simulink model "battery_fault_detection_model"  (R2024a)
settings: Solver=VariableStepAuto  StartTime=0.0  StopTime=3000  RelTol=1e-3
undefined symbols (not defined in the file or in its folder): a1, a1_1, a1_2, a1_3, a1_4, A2, a2, A2_2, A2_3, A2_4, A2_5, b1, b1_1, b1_2, b1_3, b1_4, B2, B2_2, B2_3, B2_4, B2_5, C1, C2m, C2m_2, C2m_3, C2m_4, C2m_5, Cbat, Cell, D2, D2_2, D2_3, D2_4, D2_5, dOCV, OCV, P0, Qb, R, R1, SoC0, SOC_bp, Ts
libraries: simulink x8, dspstat3 x1
settings Model: Creator=mukir  LastModifiedBy=mukir
settings DataIOCC: ReturnWorkspaceOutputs=off

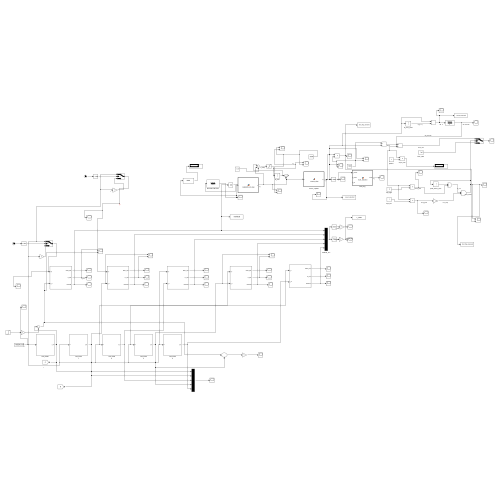
[thumbnail: Simulink's stored preview of the top-level diagram]
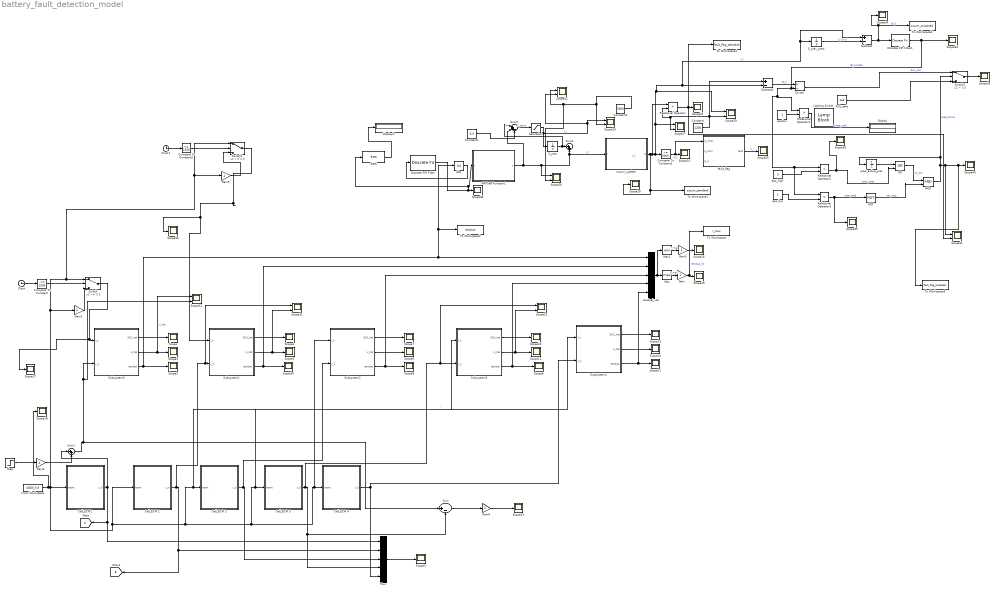
== system battery_fault_detection_model ==
  note: d_i
  note: d_i
  AND : Logic  IconShape=distinctive  AllPortsSameDT=off  OutDataTypeStr=boolean
  Abs : Abs  SaturateOnIntegerOverflow=off
  Cell_ECM 1 : Subsystem
  Cell_ECM 2 : Subsystem
  Cell_ECM 3 : Subsystem
  Cell_ECM 4 : Subsystem
  "Cell_ECM1 " : Subsystem
  Clock : Clock
  Clock1 : Clock
  Compare To Constant : simulink/Logic and Bit Operations/Compare To Constant  relop=<=  const=1500  OutDataTypeStr=boolean
  Compare To Constant1 : simulink/Logic and Bit Operations/Compare To Constant  relop=>=  const=3000  OutDataTypeStr=boolean
  Compare To Constant2 : simulink/Logic and Bit Operations/Compare To Constant  relop=<=  const=1500  OutDataTypeStr=boolean
  Constant : Constant  Value=1200
  Constant1 : Constant  Value=0.5
  Constant2 : Constant  Value=3000
  Discrete FIR Filter : DiscreteFir  Coefficients=(1/50)*ones(1,50)
  Discrete FIR Filter1 : DiscreteFir  Coefficients=ones(1,10)/10
  Display : Display
  Display2 : Display
  Divide : Product  Inputs=*/
  From Workspace : FromWorkspace  VariableName=UDDS_full  SampleTime=1
  Gain{,1..5} (6 alike) : Gain
  Goto : Goto  TagVisibility=global
  Lighting Switch : LampBlock  LabelPosition=Hide  Icon=LightingSwitch
  MATLAB Function1 : MATLAB Function  TreatAsAtomicUnit=on
  Max : MinMax  Function=max
  Max1 : MinMax
  Mux : Mux  Inputs=5
  NOT : Logic  Operator=NOT  IconShape=distinctive  AllPortsSameDT=off  OutDataTypeStr=boolean
  OR : Logic  Operator=OR  IconShape=distinctive  AllPortsSameDT=off  OutDataTypeStr=boolean
  RMS : dspstat3/RMS  run=off  directionMode=Each column  dimension=1  InputProcessing=Columns as channels (frame based)  reset_popup=None
  "RUL_safe " : Constant  Value=1e6
  Relational Operator : RelationalOperator  Operator=>  OutDataTypeStr=boolean  RndMeth=Simplest  InputSameDT=off
  Relational Operator1 : RelationalOperator  Operator=>  OutDataTypeStr=boolean  RndMeth=Simplest  InputSameDT=off
  Relational Operator2 : RelationalOperator  Operator=>  OutDataTypeStr=boolean  RndMeth=Simplest  InputSameDT=off
  Relational Operator3 : RelationalOperator  Operator=<  OutDataTypeStr=boolean  RndMeth=Simplest  InputSameDT=off
  "S_prev " : UnitDelay  SampleTime=-1  HasFrameUpgradeWarning=on
  S_prev_pred : UnitDelay  SampleTime=-1  HasFrameUpgradeWarning=on
  Saturation : Saturate  UpperLimit=inf  LowerLimit=0
  Scope{,1..11,13..18,20..21,23..25,28,30,33..40} (33 alike) : Scope
  Scope{12,19,22,26..27,29,31..32,41} (9 alike) : Scope  NumInputPorts=2
  Step : Step  Time=1500  After=0.02  SampleTime=0
  Subsystem1 : Subsystem
  Subsystem2 : Subsystem
  Subsystem3 : Subsystem
  Subsystem4 : Subsystem
  Subsystem5 : Subsystem
  Subtract : Sum  Inputs=+-
  Subtract1 : Sum  Inputs=+-
  Sum : Sum  Inputs=|+-
  Sum1 : Sum  Inputs=|++
  Sum2 : Sum  Inputs=|++
  Sum5 : Sum  Inputs=|++-
  Switch : Switch  Threshold=0.5  SaturateOnIntegerOverflow=off  InputSameDT=off
  Switch1 : Switch  Threshold=0.5  SaturateOnIntegerOverflow=off  InputSameDT=off
  Switch2 : Switch  Criteria=u2 > Threshold  Threshold=0.5  SaturateOnIntegerOverflow=off  InputSameDT=off
  To Workspace : ToWorkspace  VariableName=r_max  SaveFormat=Timeseries  SampleTime=-1
  To Workspace1 : ToWorkspace  VariableName=cusum_standard  SampleTime=-1
  To Workspace2 : ToWorkspace  VariableName=residual  SampleTime=-1
  To Workspace3 : ToWorkspace  VariableName=cusum_proposed  SaveFormat=Timeseries  SampleTime=-1
  To Workspace4 : ToWorkspace  VariableName=fault_flag_standard  SampleTime=-1
  To Workspace5 : ToWorkspace  VariableName=fault_flag_proposed  SampleTime=-1
  "cusum_update " : MATLAB Function  TreatAsAtomicUnit=on
  eps_high : Constant  Value=3
  eps_low : Constant
  "epsilon " : Constant
  fault_flag : MATLAB Function  TreatAsAtomicUnit=on
  "pred_active_prev " : UnitDelay  SampleTime=-1  HasFrameUpgradeWarning=on
  "residual_vec " : Mux  Inputs=5
  tag scope: B=global
  wires:
  Gain2/1 -> Sum1/2
  Step/1 -> Gain2/1
  Subsystem5/1(SOC_hat) -> Scope/1
  Subsystem5/3(residual) -> To Workspace2/1, Abs/1, "residual_vec "/1, Scope2/1
  Cell_ECM 1/1(y_k) -> Scope31/1, Subsystem1/2(y_k), [B], Mux/2
  Cell_ECM 2/1(y_k) -> Subsystem2/2(y_k), Mux/3
  Cell_ECM 4/1(y_k) -> Subsystem4/2(y_k), Mux/5
  Mux/1 -> Scope3/1
  Subsystem1/2(U_hat) -> Scope31/2, Scope5/1
  Subsystem1/1(SOC_hat) -> Scope4/1
  Subsystem2/3(residual) -> "residual_vec "/3, Scope8/1
  Subsystem2/1(SOC_hat) -> Scope7/1
  Subsystem3/3(residual) -> Scope6/1, "residual_vec "/4
  Subsystem3/1(SOC_hat) -> Scope10/1
  Subsystem4/3(residual) -> Scope21/1, "residual_vec "/5
  Subsystem4/2(U_hat) -> Scope14/1
  Subsystem4/1(SOC_hat) -> Scope13/1
  "residual_vec "/1 -> Max1/1, Max/1
  Max/1 -> Gain/1  "r_max"
  Clock/1 -> Compare To Constant/1
  Gain1/1 -> Switch/3
  Compare To Constant/1 -> Switch/2
  Max1/1 -> Gain3/1  "r_max"
  Gain3/1 -> Scope16/1
  Switch/1 -> Scope17/1, Subsystem5/1(I_k)
  Gain/1 -> Scope15/1, To Workspace/1  "residual_hp"
  Subsystem5/2(U_hat) -> Scope22/1, Scope1/1  "U_hat"
  Sum1/1 -> Scope22/2, Subsystem5/2(y_k), Sum/1
  Sum/1 -> Gain4/1
  Gain4/1 -> Scope23/1
  RMS/1 -> Display2/1
  Abs/1 -> Discrete FIR Filter/1
  Constant1/1 -> Sum5/3
  fault_flag/1(fault) -> Scope25/1  "s_i"
  Constant2/1 -> Scope19/2, Scope26/2, Scope32/1
  Sum5/1 -> Saturation/1  "S_temp"
  Compare To Constant1/1 -> fault_flag/1(d_umax), Scope24/1
  Constant/1 -> Subtract1/1, Scope29/2, Scope27/2, Relational Operator/2
  Discrete FIR Filter/1 -> RMS/1, MATLAB Function1/1(r), Scope36/1
  "S_prev "/1 -> Sum5/1, Sum2/1
  Saturation/1 -> Scope19/1, Scope32/2, "S_prev "/1  "s_i"
  Relational Operator/1 -> To Workspace4/1, Scope41/2, Scope37/1
  MATLAB Function1/1(s) -> Sum5/2, Scope26/1, "cusum_update "/1(r), Sum2/2  "s_i"
  "cusum_update "/1(S) -> To Workspace1/1, Scope28/1, Relational Operator/1, Subtract/1, S_prev_pred/1, Subtract1/2, Scope29/1, Scope27/1, Compare To Constant1/1  "s_i"
  "Cell_ECM1 "/1(y_k) -> Goto/1, Mux/1, Sum1/1
  Subsystem2/2(U_hat) -> Scope9/1
  Subsystem3/2(U_hat) -> Scope12/2, Scope11/1
  Cell_ECM 3/1(y_k) -> Scope12/1, Subsystem3/2(y_k), Sum/2, Mux/4
  Gain5/1 -> Switch1/3
  From Workspace/1 -> Scope18/1, Cell_ECM 1/1(Inport), Subsystem2/1(I_k), Cell_ECM 2/1(Inport), Subsystem3/1(I_k), Cell_ECM 3/1(Inport), Subsystem4/1(I_k), Cell_ECM 4/1(Inport), "Cell_ECM1 "/1(Inport), Switch1/1, Gain5/1, Switch/1, Gain1/1  "I"
  Compare To Constant2/1 -> Switch1/2
  Switch1/1 -> Subsystem1/1(I_k), Scope30/1
  Clock1/1 -> Compare To Constant2/1
  Subsystem1/3(residual) -> Scope20/1, "residual_vec "/2
  S_prev_pred/1 -> Subtract/2  "S_(k−1)"
  Subtract/1 -> Discrete FIR Filter1/1, To Workspace3/1, Scope34/1  "dS_k"
  Discrete FIR Filter1/1 -> Relational Operator3/1, Relational Operator2/1, Relational Operator1/1, Divide/2, Scope33/1  "dS_smooth"
  Subtract1/1 -> Divide/1  "dS_k"
  "epsilon "/1 -> Relational Operator1/2
  Relational Operator1/1 -> Display/1  "slope_valid"
  Divide/1 -> Switch2/1  "RUL_raw"
  "RUL_safe "/1 -> Switch2/3
  Switch2/1 -> Scope35/1
  eps_high/1 -> Relational Operator2/2
  Relational Operator2/1 -> Scope38/1, OR/2  "start_pred"
  eps_low/1 -> Relational Operator3/2
  Relational Operator3/1 -> Scope39/1, NOT/1  "stop_pred"
  "pred_active_prev "/1 -> OR/1
  OR/1 -> AND/1  "or_out"
  NOT/1 -> AND/2  "not_stop"
  AND/1 -> To Workspace5/1, Scope40/1, Scope41/1, Switch2/2, "pred_active_prev "/1  "pred_active"

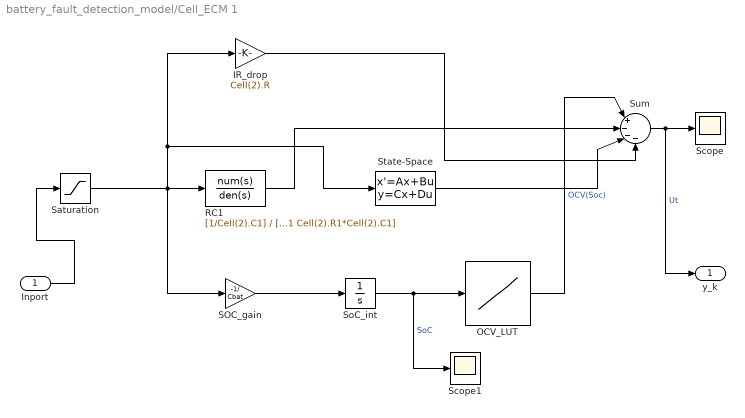
== system battery_fault_detection_model/Cell_ECM 1 ==
  Inport : Inport
  IR_drop : Gain  Gain=Cell(2).R
  OCV_LUT : Lookup_n-D  NumberOfTableDimensions=1  BreakpointsForDimension1=SOC_bp  Table=OCV  InternalRulePriority=Speed  RndMeth=Simplest
  RC1 : TransferFcn  Numerator=[1/Cell(2).C1]  Denominator=[1 Cell(2).R1*Cell(2).C1]
  SOC_gain : Gain  Gain=-1/ Cbat
  Saturation : Saturate  UpperLimit=12  LowerLimit=-6
  Scope : Scope
  Scope1 : Scope
  SoC_int : Integrator  InitialCondition=SoC0
  State-Space : StateSpace  A=A2_2  B=B2_2  C=C2m_2  D=D2_2  InitialCondition=0
  Sum : Sum  Inputs=|+---
  y_k : Outport
  wires:
  IR_drop/1 -> Sum/4
  RC1/1 -> Sum/2
  Saturation/1 -> SOC_gain/1, State-Space/1, IR_drop/1, RC1/1
  SOC_gain/1 -> SoC_int/1
  OCV_LUT/1 -> Sum/1  "OCV(Soc)"
  SoC_int/1 -> Scope1/1, OCV_LUT/1  "SoC"
  Sum/1 -> y_k/1, Scope/1  "Ut"
  State-Space/1 -> Sum/3
  Inport/1 -> Saturation/1

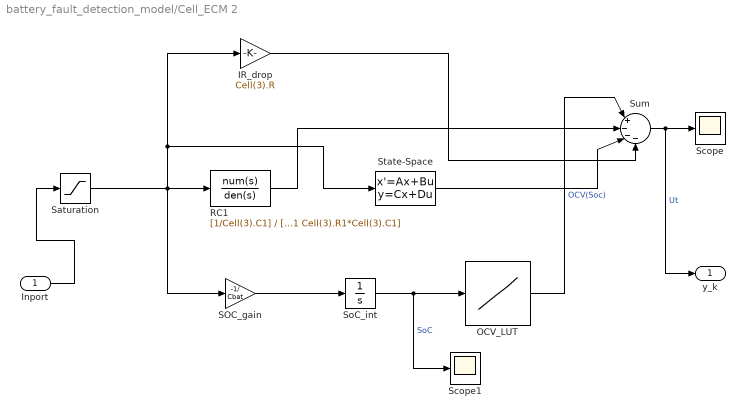
== system battery_fault_detection_model/Cell_ECM 2 ==
  Inport : Inport
  IR_drop : Gain  Gain=Cell(3).R
  OCV_LUT : Lookup_n-D  NumberOfTableDimensions=1  BreakpointsForDimension1=SOC_bp  Table=OCV  InternalRulePriority=Speed  RndMeth=Simplest
  RC1 : TransferFcn  Numerator=[1/Cell(3).C1]  Denominator=[1 Cell(3).R1*Cell(3).C1]
  SOC_gain : Gain  Gain=-1/ Cbat
  Saturation : Saturate  UpperLimit=12  LowerLimit=-6
  Scope : Scope
  Scope1 : Scope
  SoC_int : Integrator  InitialCondition=SoC0
  State-Space : StateSpace  A=A2_3  B=B2_3  C=C2m_3  D=D2_3  InitialCondition=0
  Sum : Sum  Inputs=|+---
  y_k : Outport
  wires:
  IR_drop/1 -> Sum/4
  RC1/1 -> Sum/2
  Saturation/1 -> SOC_gain/1, State-Space/1, IR_drop/1, RC1/1
  SOC_gain/1 -> SoC_int/1
  OCV_LUT/1 -> Sum/1  "OCV(Soc)"
  SoC_int/1 -> Scope1/1, OCV_LUT/1  "SoC"
  Sum/1 -> y_k/1, Scope/1  "Ut"
  State-Space/1 -> Sum/3
  Inport/1 -> Saturation/1

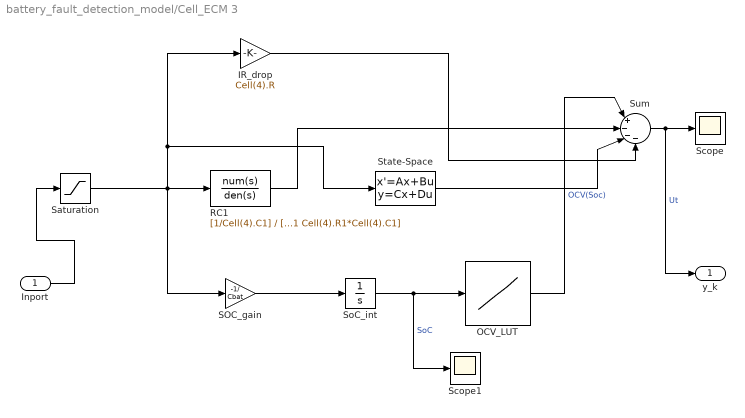
== system battery_fault_detection_model/Cell_ECM 3 ==
  Inport : Inport
  IR_drop : Gain  Gain=Cell(4).R
  OCV_LUT : Lookup_n-D  NumberOfTableDimensions=1  BreakpointsForDimension1=SOC_bp  Table=OCV  InternalRulePriority=Speed  RndMeth=Simplest
  RC1 : TransferFcn  Numerator=[1/Cell(4).C1]  Denominator=[1 Cell(4).R1*Cell(4).C1]
  SOC_gain : Gain  Gain=-1/ Cbat
  Saturation : Saturate  UpperLimit=12  LowerLimit=-6
  Scope : Scope
  Scope1 : Scope
  SoC_int : Integrator  InitialCondition=SoC0
  State-Space : StateSpace  A=A2_4  B=B2_4  C=C2m_4  D=D2_4  InitialCondition=0
  Sum : Sum  Inputs=|+---
  y_k : Outport
  wires:
  IR_drop/1 -> Sum/4
  RC1/1 -> Sum/2
  Saturation/1 -> SOC_gain/1, State-Space/1, IR_drop/1, RC1/1
  SOC_gain/1 -> SoC_int/1
  OCV_LUT/1 -> Sum/1  "OCV(Soc)"
  SoC_int/1 -> Scope1/1, OCV_LUT/1  "SoC"
  Sum/1 -> y_k/1, Scope/1  "Ut"
  State-Space/1 -> Sum/3
  Inport/1 -> Saturation/1

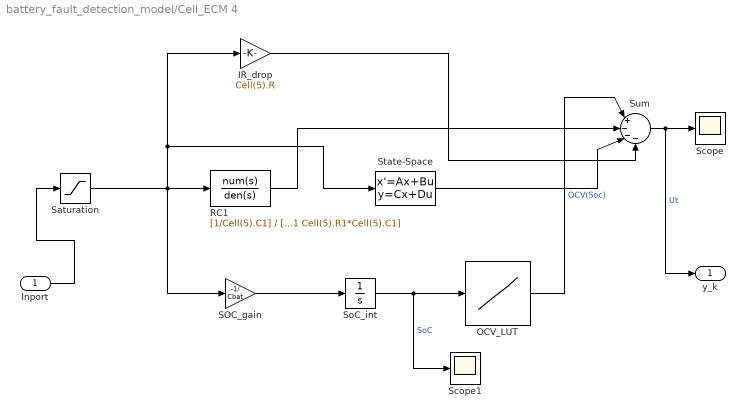
== system battery_fault_detection_model/Cell_ECM 4 ==
  Inport : Inport
  IR_drop : Gain  Gain=Cell(5).R
  OCV_LUT : Lookup_n-D  NumberOfTableDimensions=1  BreakpointsForDimension1=SOC_bp  Table=OCV  InternalRulePriority=Speed  RndMeth=Simplest
  RC1 : TransferFcn  Numerator=[1/Cell(5).C1]  Denominator=[1 Cell(5).R1*Cell(5).C1]
  SOC_gain : Gain  Gain=-1/ Cbat
  Saturation : Saturate  UpperLimit=12  LowerLimit=-6
  Scope : Scope
  Scope1 : Scope
  SoC_int : Integrator  InitialCondition=SoC0
  State-Space : StateSpace  A=A2_5  B=B2_5  C=C2m_5  D=D2_5  InitialCondition=0
  Sum : Sum  Inputs=|+---
  y_k : Outport
  wires:
  IR_drop/1 -> Sum/4
  RC1/1 -> Sum/2
  Saturation/1 -> SOC_gain/1, State-Space/1, IR_drop/1, RC1/1
  SOC_gain/1 -> SoC_int/1
  OCV_LUT/1 -> Sum/1  "OCV(Soc)"
  SoC_int/1 -> Scope1/1, OCV_LUT/1  "SoC"
  Sum/1 -> y_k/1, Scope/1  "Ut"
  State-Space/1 -> Sum/3
  Inport/1 -> Saturation/1

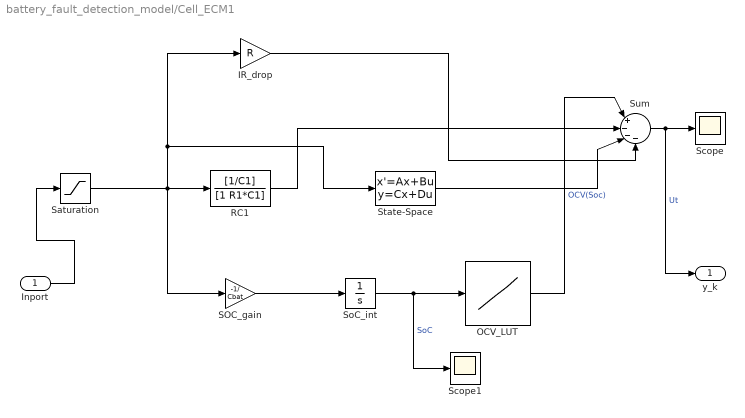
== system battery_fault_detection_model/Cell_ECM1  ==
  Inport : Inport
  IR_drop : Gain  Gain=R
  OCV_LUT : Lookup_n-D  NumberOfTableDimensions=1  BreakpointsForDimension1=SOC_bp  Table=OCV  InternalRulePriority=Speed  RndMeth=Simplest
  RC1 : TransferFcn  Numerator=[1/C1]  Denominator=[1 R1*C1]
  SOC_gain : Gain  Gain=-1/ Cbat
  Saturation : Saturate  UpperLimit=12  LowerLimit=-6
  Scope : Scope
  Scope1 : Scope
  SoC_int : Integrator  InitialCondition=SoC0
  State-Space : StateSpace  A=A2  B=B2  C=C2m  D=D2  InitialCondition=0
  Sum : Sum  Inputs=|+---
  y_k : Outport
  wires:
  IR_drop/1 -> Sum/4
  RC1/1 -> Sum/2
  Saturation/1 -> SOC_gain/1, State-Space/1, IR_drop/1, RC1/1
  SOC_gain/1 -> SoC_int/1
  OCV_LUT/1 -> Sum/1  "OCV(Soc)"
  SoC_int/1 -> Scope1/1, OCV_LUT/1  "SoC"
  Sum/1 -> y_k/1, Scope/1  "Ut"
  State-Space/1 -> Sum/3
  Inport/1 -> Saturation/1

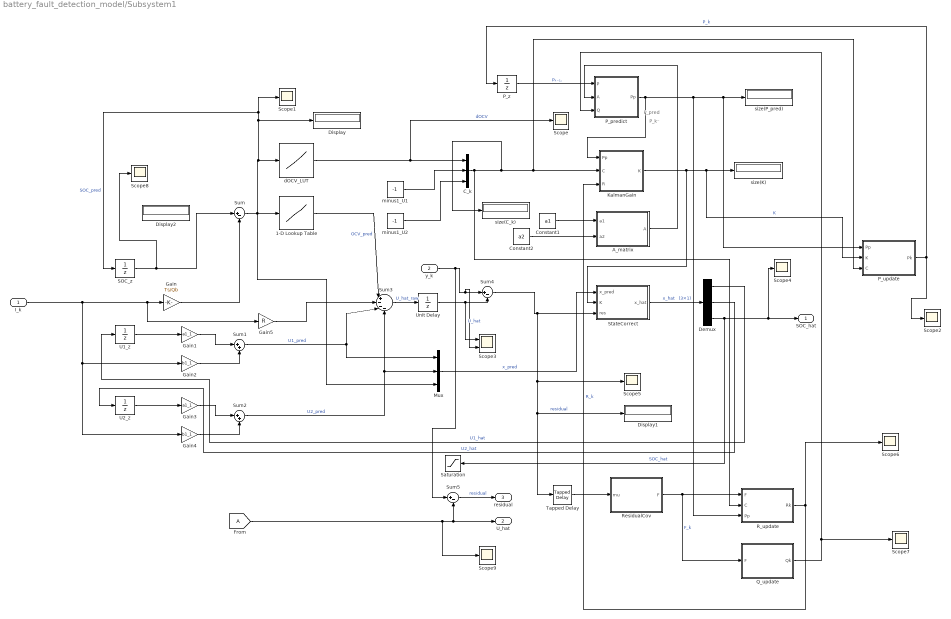
== system battery_fault_detection_model/Subsystem1 ==
  note: P_pred
  note: P_k⁻
  I_k : Inport
  y_k : Inport  Port=2
  1-D Lookup Table : Lookup_n-D  NumberOfTableDimensions=1  BreakpointsForDimension1=SOC_bp  Table=OCV  InternalRulePriority=Speed  RndMeth=Simplest
  A_matrix : MATLAB Function  TreatAsAtomicUnit=on
  "C_k " : Mux  Inputs=3
  Constant1 : Constant  Value=a1
  Constant2 : Constant  Value=a2
  Demux : Demux  Outputs=3
  Display : Display
  Display1 : Display
  Display2 : Display
  From : From  TagVisibility=global
  Gain : Gain  Gain=Ts/Qb
  Gain1 : Gain  Gain=a1_1
  Gain2 : Gain  Gain=b1_1
  Gain3 : Gain  Gain=a1_1
  Gain4 : Gain  Gain=b1_1
  Gain5 : Gain  Gain=R
  KalmanGain : MATLAB Function  TreatAsAtomicUnit=on
  Mux : Mux  Inputs=3
  P_predict : MATLAB Function  TreatAsAtomicUnit=on
  "P_update " : MATLAB Function  TreatAsAtomicUnit=on
  P_z : UnitDelay  InitialCondition=P0  SampleTime=-1  HasFrameUpgradeWarning=on
  Q_update : MATLAB Function  TreatAsAtomicUnit=on
  R_update : MATLAB Function  TreatAsAtomicUnit=on
  ResidualCov : MATLAB Function  TreatAsAtomicUnit=on
  SOC_z : UnitDelay  InitialCondition=0.6  SampleTime=-1  HasFrameUpgradeWarning=on
  Saturation : Saturate  UpperLimit=1  LowerLimit=0
  Scope{,1..2,4..9} (9 alike) : Scope
  Scope3 : Scope  NumInputPorts=2
  "StateCorrect " : MATLAB Function  TreatAsAtomicUnit=on
  Sum : Sum  Inputs=|+-
  Sum1 : Sum  Inputs=|++
  Sum2 : Sum  Inputs=|++
  Sum3 : Sum  Inputs=|+---
  Sum4 : Sum  Inputs=|+-
  Sum5 : Sum  Inputs=|+-
  Tapped Delay : simulink/Discrete/Tapped Delay  vinit=0.0  samptime=-1  NumDelays=20  DelayOrder=Newest  includeCurrent=on
  U1_z : UnitDelay  SampleTime=-1  HasFrameUpgradeWarning=on
  U2_z : UnitDelay  SampleTime=-1  HasFrameUpgradeWarning=on
  Unit Delay : UnitDelay  InitialCondition=3.33  SampleTime=-1  HasFrameUpgradeWarning=on
  "dOCV_LUT " : Lookup_n-D  NumberOfTableDimensions=1  BreakpointsForDimension1=SOC_bp  Table=dOCV  InternalRulePriority=Speed  RndMeth=Simplest
  minus1_U1 : Constant  Value=-1
  minus1_U2 : Constant  Value=-1
  size(C_k) : Display
  size(K) : Display
  size(P_pred) : Display
  SOC_hat : Outport
  U_hat : Outport  Port=2
  residual : Outport  Port=3
  wires:
  Gain/1 -> Sum/2
  Sum/1 -> Mux/3, Display/1, SOC_z/1, Scope1/1, "dOCV_LUT "/1, 1-D Lookup Table/1  "SOC_pred"
  U1_z/1 -> Gain1/1
  Gain1/1 -> Sum1/1
  Gain2/1 -> Sum1/2
  Sum1/1 -> Sum3/3, Mux/1  "U1_pred"
  Sum2/1 -> Mux/2, Sum3/4  "U2_pred"
  Gain4/1 -> Sum2/2
  U2_z/1 -> Gain3/1
  Gain3/1 -> Sum2/1
  1-D Lookup Table/1 -> Sum3/1  "OCV_pred"
  Gain5/1 -> Sum3/2
  Sum3/1 -> Unit Delay/1  "U_hat_raw"
  Unit Delay/1 -> Scope3/1, Sum4/2  "U_hat"
  y_k/1 -> Sum5/1, Scope3/2, Sum4/1
  Sum4/1 -> Scope5/1, Display1/1, Tapped Delay/1, "StateCorrect "/3(res)  "residual"
  "dOCV_LUT "/1 -> Scope/1, "C_k "/1  "dOCV"
  minus1_U1/1 -> "C_k "/2
  minus1_U2/1 -> "C_k "/3
  I_k/1 -> Gain4/1, Gain2/1, Gain5/1, Gain/1
  P_z/1 -> P_predict/1(P)  "Pₖ₋₁."
  P_predict/1(Pp) -> "P_update "/1(Pp), size(P_pred)/1, R_update/3(Pp), KalmanGain/1(Pp)
  "C_k "/1 -> size(C_k)/1, "P_update "/3(C), KalmanGain/2(C), R_update/2(C)
  Constant1/1 -> A_matrix/1(a1)
  Constant2/1 -> A_matrix/2(a2)
  A_matrix/1(A) -> P_predict/2(A)
  Q_update/1(Qk) -> Scope7/1, P_predict/3(Q)
  KalmanGain/1(K) -> "StateCorrect "/2(K), "P_update "/2(K), size(K)/1  "K"
  Mux/1 -> "StateCorrect "/1(x_pred)  "x_pred"
  "StateCorrect "/1(x_hat) -> Demux/1  "x_hat   (3×1)"
  Demux/1 -> U1_z/1  "U1_hat"
  Demux/2 -> U2_z/1  "U2_hat"
  Demux/3 -> Saturation/1, Scope4/1, SOC_hat/1  "SOC_hat"
  Tapped Delay/1 -> ResidualCov/1(mu)
  ResidualCov/1(F) -> Q_update/1(F), R_update/1(F)  "F_k"
  R_update/1(Rk) -> KalmanGain/3(R), Scope6/1  "R_k"
  "P_update "/1(Pk) -> Scope2/1, P_z/1  "P_k"
  SOC_z/1 -> Scope8/1, Sum/1
  From/1 -> Scope9/1, U_hat/1, Sum5/2
  Sum5/1 -> residual/1  "residual"

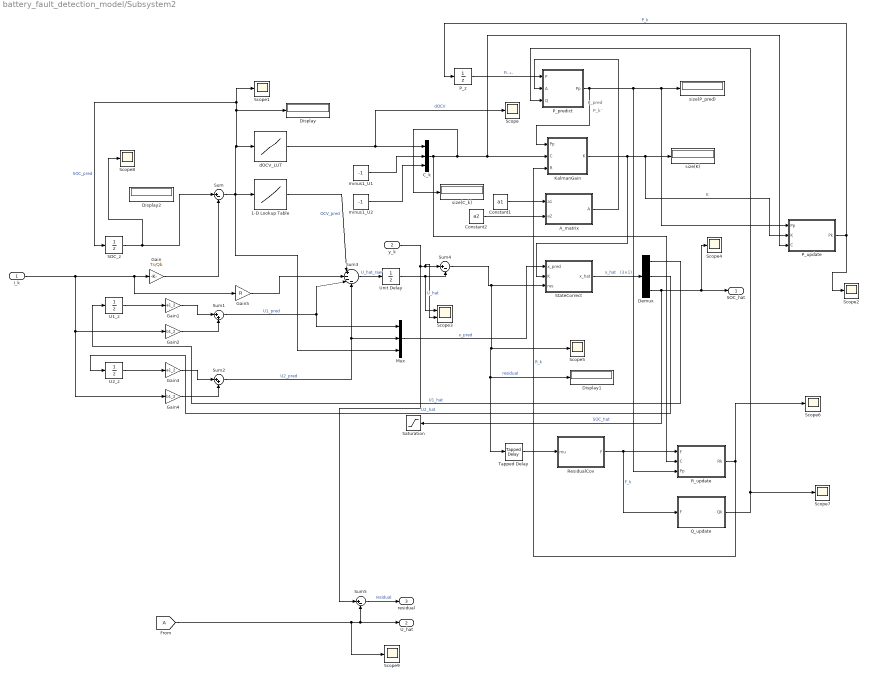
== system battery_fault_detection_model/Subsystem2 ==
  note: P_pred
  note: P_k⁻
  I_k : Inport
  y_k : Inport  Port=2
  1-D Lookup Table : Lookup_n-D  NumberOfTableDimensions=1  BreakpointsForDimension1=SOC_bp  Table=OCV  InternalRulePriority=Speed  RndMeth=Simplest
  A_matrix : MATLAB Function  TreatAsAtomicUnit=on
  "C_k " : Mux  Inputs=3
  Constant1 : Constant  Value=a1
  Constant2 : Constant  Value=a2
  Demux : Demux  Outputs=3
  Display : Display
  Display1 : Display
  Display2 : Display
  From : From  TagVisibility=global
  Gain : Gain  Gain=Ts/Qb
  Gain1 : Gain  Gain=a1_2
  Gain2 : Gain  Gain=b1_2
  Gain3 : Gain  Gain=a1_2
  Gain4 : Gain  Gain=b1_2
  Gain5 : Gain  Gain=R
  KalmanGain : MATLAB Function  TreatAsAtomicUnit=on
  Mux : Mux  Inputs=3
  P_predict : MATLAB Function  TreatAsAtomicUnit=on
  "P_update " : MATLAB Function  TreatAsAtomicUnit=on
  P_z : UnitDelay  InitialCondition=P0  SampleTime=-1  HasFrameUpgradeWarning=on
  Q_update : MATLAB Function  TreatAsAtomicUnit=on
  R_update : MATLAB Function  TreatAsAtomicUnit=on
  ResidualCov : MATLAB Function  TreatAsAtomicUnit=on
  SOC_z : UnitDelay  InitialCondition=0.6  SampleTime=-1  HasFrameUpgradeWarning=on
  Saturation : Saturate  UpperLimit=1  LowerLimit=0
  Scope{,1..2,4..9} (9 alike) : Scope
  Scope3 : Scope  NumInputPorts=2
  "StateCorrect " : MATLAB Function  TreatAsAtomicUnit=on
  Sum : Sum  Inputs=|+-
  Sum1 : Sum  Inputs=|++
  Sum2 : Sum  Inputs=|++
  Sum3 : Sum  Inputs=|+---
  Sum4 : Sum  Inputs=|+-
  Sum5 : Sum  Inputs=|+-
  Tapped Delay : simulink/Discrete/Tapped Delay  vinit=0.0  samptime=-1  NumDelays=20  DelayOrder=Newest  includeCurrent=on
  U1_z : UnitDelay  SampleTime=-1  HasFrameUpgradeWarning=on
  U2_z : UnitDelay  SampleTime=-1  HasFrameUpgradeWarning=on
  Unit Delay : UnitDelay  InitialCondition=3.33  SampleTime=-1  HasFrameUpgradeWarning=on
  "dOCV_LUT " : Lookup_n-D  NumberOfTableDimensions=1  BreakpointsForDimension1=SOC_bp  Table=dOCV  InternalRulePriority=Speed  RndMeth=Simplest
  minus1_U1 : Constant  Value=-1
  minus1_U2 : Constant  Value=-1
  size(C_k) : Display
  size(K) : Display
  size(P_pred) : Display
  SOC_hat : Outport
  U_hat : Outport  Port=2
  residual : Outport  Port=3
  wires:
  Gain/1 -> Sum/2
  Sum/1 -> Mux/3, Display/1, SOC_z/1, Scope1/1, "dOCV_LUT "/1, 1-D Lookup Table/1  "SOC_pred"
  U1_z/1 -> Gain1/1
  Gain1/1 -> Sum1/1
  Gain2/1 -> Sum1/2
  Sum1/1 -> Sum3/3, Mux/1  "U1_pred"
  Sum2/1 -> Mux/2, Sum3/4  "U2_pred"
  Gain4/1 -> Sum2/2
  U2_z/1 -> Gain3/1
  Gain3/1 -> Sum2/1
  1-D Lookup Table/1 -> Sum3/1  "OCV_pred"
  Gain5/1 -> Sum3/2
  Sum3/1 -> Unit Delay/1  "U_hat_raw"
  Unit Delay/1 -> Scope3/1, Sum4/2  "U_hat"
  Sum4/1 -> Scope5/1, Display1/1, Tapped Delay/1, "StateCorrect "/3(res)  "residual"
  "dOCV_LUT "/1 -> Scope/1, "C_k "/1  "dOCV"
  minus1_U1/1 -> "C_k "/2
  minus1_U2/1 -> "C_k "/3
  I_k/1 -> Gain4/1, Gain2/1, Gain5/1, Gain/1
  P_z/1 -> P_predict/1(P)  "Pₖ₋₁."
  P_predict/1(Pp) -> "P_update "/1(Pp), size(P_pred)/1, R_update/3(Pp), KalmanGain/1(Pp)
  "C_k "/1 -> size(C_k)/1, "P_update "/3(C), KalmanGain/2(C), R_update/2(C)
  Constant1/1 -> A_matrix/1(a1)
  Constant2/1 -> A_matrix/2(a2)
  A_matrix/1(A) -> P_predict/2(A)
  Q_update/1(Qk) -> Scope7/1, P_predict/3(Q)
  KalmanGain/1(K) -> "StateCorrect "/2(K), "P_update "/2(K), size(K)/1  "K"
  Mux/1 -> "StateCorrect "/1(x_pred)  "x_pred"
  "StateCorrect "/1(x_hat) -> Demux/1  "x_hat   (3×1)"
  Demux/1 -> U1_z/1  "U1_hat"
  Demux/2 -> U2_z/1  "U2_hat"
  Demux/3 -> Saturation/1, Scope4/1, SOC_hat/1  "SOC_hat"
  Tapped Delay/1 -> ResidualCov/1(mu)
  ResidualCov/1(F) -> Q_update/1(F), R_update/1(F)  "F_k"
  R_update/1(Rk) -> KalmanGain/3(R), Scope6/1  "R_k"
  "P_update "/1(Pk) -> Scope2/1, P_z/1  "P_k"
  SOC_z/1 -> Scope8/1, Sum/1
  Sum5/1 -> residual/1  "residual"
  From/1 -> Scope9/1, U_hat/1, Sum5/2
  y_k/1 -> Sum5/1, Scope3/2, Sum4/1

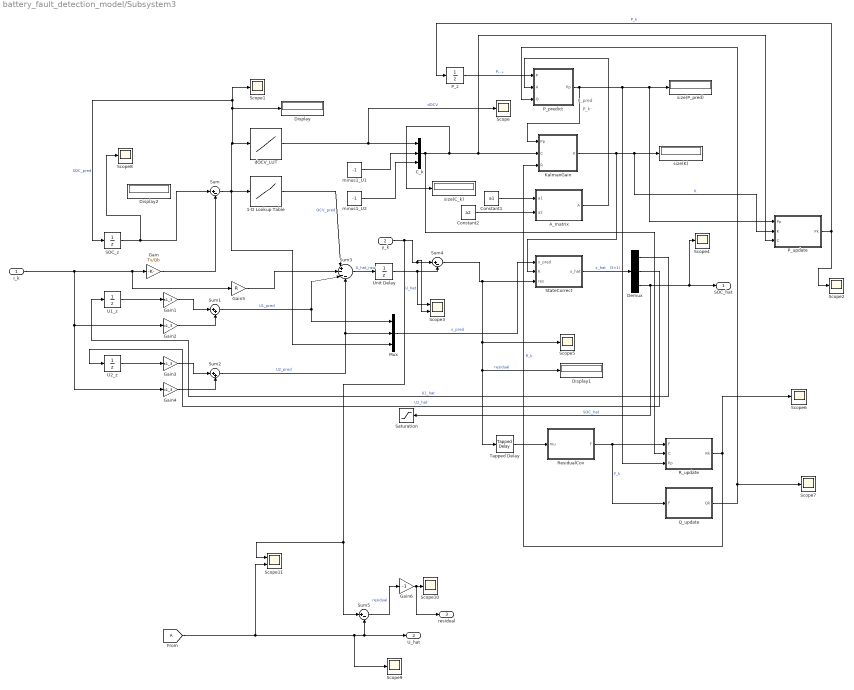
== system battery_fault_detection_model/Subsystem3 ==
  note: P_pred
  note: P_k⁻
  I_k : Inport
  y_k : Inport  Port=2
  1-D Lookup Table : Lookup_n-D  NumberOfTableDimensions=1  BreakpointsForDimension1=SOC_bp  Table=OCV  InternalRulePriority=Speed  RndMeth=Simplest
  A_matrix : MATLAB Function  TreatAsAtomicUnit=on
  "C_k " : Mux  Inputs=3
  Constant1 : Constant  Value=a1
  Constant2 : Constant  Value=a2
  Demux : Demux  Outputs=3
  Display : Display
  Display1 : Display
  Display2 : Display
  From : From  TagVisibility=global
  Gain : Gain  Gain=Ts/Qb
  Gain1 : Gain  Gain=a1_3
  Gain2 : Gain  Gain=b1_3
  Gain3 : Gain  Gain=a1_3
  Gain4 : Gain  Gain=b1_3
  Gain5 : Gain  Gain=R
  Gain6 : Gain  Gain=-1
  KalmanGain : MATLAB Function  TreatAsAtomicUnit=on
  Mux : Mux  Inputs=3
  P_predict : MATLAB Function  TreatAsAtomicUnit=on
  "P_update " : MATLAB Function  TreatAsAtomicUnit=on
  P_z : UnitDelay  InitialCondition=P0  SampleTime=-1  HasFrameUpgradeWarning=on
  Q_update : MATLAB Function  TreatAsAtomicUnit=on
  R_update : MATLAB Function  TreatAsAtomicUnit=on
  ResidualCov : MATLAB Function  TreatAsAtomicUnit=on
  SOC_z : UnitDelay  InitialCondition=0.6  SampleTime=-1  HasFrameUpgradeWarning=on
  Saturation : Saturate  UpperLimit=1  LowerLimit=0
  Scope{,1..2,4..10} (10 alike) : Scope
  Scope11 : Scope  NumInputPorts=2
  Scope3 : Scope  NumInputPorts=2
  "StateCorrect " : MATLAB Function  TreatAsAtomicUnit=on
  Sum : Sum  Inputs=|+-
  Sum1 : Sum  Inputs=|++
  Sum2 : Sum  Inputs=|++
  Sum3 : Sum  Inputs=|+---
  Sum4 : Sum  Inputs=|+-
  Sum5 : Sum  Inputs=|+-
  Tapped Delay : simulink/Discrete/Tapped Delay  vinit=0.0  samptime=-1  NumDelays=20  DelayOrder=Newest  includeCurrent=on
  U1_z : UnitDelay  SampleTime=-1  HasFrameUpgradeWarning=on
  U2_z : UnitDelay  SampleTime=-1  HasFrameUpgradeWarning=on
  Unit Delay : UnitDelay  InitialCondition=3.33  SampleTime=-1  HasFrameUpgradeWarning=on
  "dOCV_LUT " : Lookup_n-D  NumberOfTableDimensions=1  BreakpointsForDimension1=SOC_bp  Table=dOCV  InternalRulePriority=Speed  RndMeth=Simplest
  minus1_U1 : Constant  Value=-1
  minus1_U2 : Constant  Value=-1
  size(C_k) : Display
  size(K) : Display
  size(P_pred) : Display
  SOC_hat : Outport
  U_hat : Outport  Port=2
  residual : Outport  Port=3
  wires:
  Gain/1 -> Sum/2
  Sum/1 -> Mux/3, Display/1, SOC_z/1, Scope1/1, "dOCV_LUT "/1, 1-D Lookup Table/1  "SOC_pred"
  U1_z/1 -> Gain1/1
  Gain1/1 -> Sum1/1
  Gain2/1 -> Sum1/2
  Sum1/1 -> Sum3/3, Mux/1  "U1_pred"
  Sum2/1 -> Mux/2, Sum3/4  "U2_pred"
  Gain4/1 -> Sum2/2
  U2_z/1 -> Gain3/1
  Gain3/1 -> Sum2/1
  1-D Lookup Table/1 -> Sum3/1  "OCV_pred"
  Gain5/1 -> Sum3/2
  Sum3/1 -> Unit Delay/1  "U_hat_raw"
  Unit Delay/1 -> Scope3/1, Sum4/2  "U_hat"
  Sum4/1 -> Scope5/1, Display1/1, Tapped Delay/1, "StateCorrect "/3(res)  "residual"
  "dOCV_LUT "/1 -> Scope/1, "C_k "/1  "dOCV"
  minus1_U1/1 -> "C_k "/2
  minus1_U2/1 -> "C_k "/3
  I_k/1 -> Gain4/1, Gain2/1, Gain5/1, Gain/1
  P_z/1 -> P_predict/1(P)  "Pₖ₋₁."
  P_predict/1(Pp) -> "P_update "/1(Pp), size(P_pred)/1, R_update/3(Pp), KalmanGain/1(Pp)
  "C_k "/1 -> size(C_k)/1, "P_update "/3(C), KalmanGain/2(C), R_update/2(C)
  Constant1/1 -> A_matrix/1(a1)
  Constant2/1 -> A_matrix/2(a2)
  A_matrix/1(A) -> P_predict/2(A)
  Q_update/1(Qk) -> Scope7/1, P_predict/3(Q)
  KalmanGain/1(K) -> "StateCorrect "/2(K), "P_update "/2(K), size(K)/1  "K"
  Mux/1 -> "StateCorrect "/1(x_pred)  "x_pred"
  "StateCorrect "/1(x_hat) -> Demux/1  "x_hat   (3×1)"
  Demux/1 -> U1_z/1  "U1_hat"
  Demux/2 -> U2_z/1  "U2_hat"
  Demux/3 -> Saturation/1, Scope4/1, SOC_hat/1  "SOC_hat"
  Tapped Delay/1 -> ResidualCov/1(mu)
  ResidualCov/1(F) -> Q_update/1(F), R_update/1(F)  "F_k"
  R_update/1(Rk) -> KalmanGain/3(R), Scope6/1  "R_k"
  "P_update "/1(Pk) -> Scope2/1, P_z/1  "P_k"
  SOC_z/1 -> Scope8/1, Sum/1
  y_k/1 -> Scope11/1, Sum5/1, Scope3/2, Sum4/1
  Sum5/1 -> Gain6/1  "residual"
  From/1 -> Scope9/1, U_hat/1, Sum5/2, Scope11/2
  Gain6/1 -> residual/1, Scope10/1

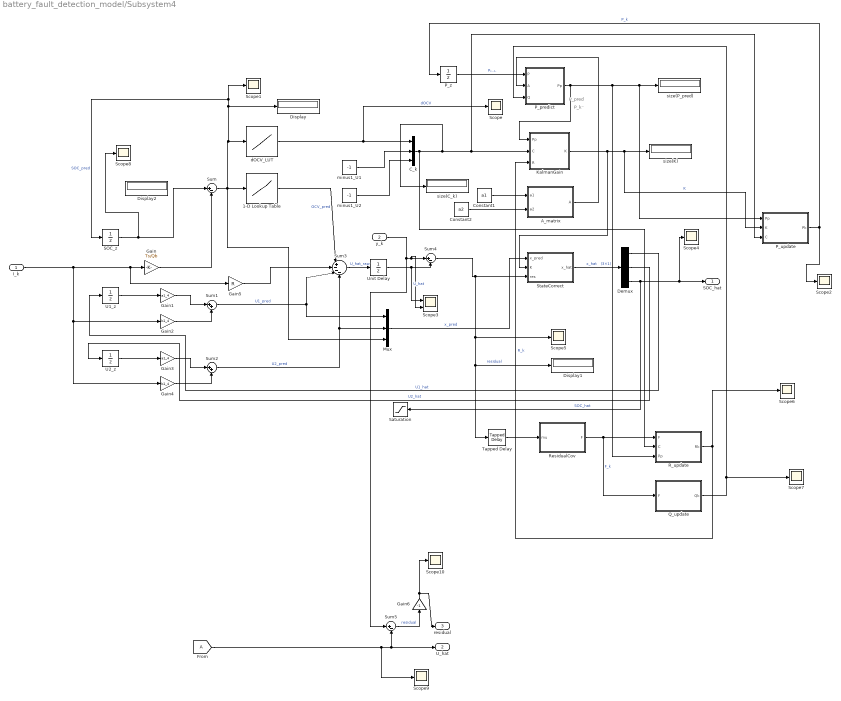
== system battery_fault_detection_model/Subsystem4 ==
  note: P_pred
  note: P_k⁻
  I_k : Inport
  y_k : Inport  Port=2
  1-D Lookup Table : Lookup_n-D  NumberOfTableDimensions=1  BreakpointsForDimension1=SOC_bp  Table=OCV  InternalRulePriority=Speed  RndMeth=Simplest
  A_matrix : MATLAB Function  TreatAsAtomicUnit=on
  "C_k " : Mux  Inputs=3
  Constant1 : Constant  Value=a1
  Constant2 : Constant  Value=a2
  Demux : Demux  Outputs=3
  Display : Display
  Display1 : Display
  Display2 : Display
  From : From  TagVisibility=global
  Gain : Gain  Gain=Ts/Qb
  Gain1 : Gain  Gain=a1_4
  Gain2 : Gain  Gain=b1_4
  Gain3 : Gain  Gain=a1_4
  Gain4 : Gain  Gain=b1_4
  Gain5 : Gain  Gain=R
  Gain6 : Gain  Gain=-1
  KalmanGain : MATLAB Function  TreatAsAtomicUnit=on
  Mux : Mux  Inputs=3
  P_predict : MATLAB Function  TreatAsAtomicUnit=on
  "P_update " : MATLAB Function  TreatAsAtomicUnit=on
  P_z : UnitDelay  InitialCondition=P0  SampleTime=-1  HasFrameUpgradeWarning=on
  Q_update : MATLAB Function  TreatAsAtomicUnit=on
  R_update : MATLAB Function  TreatAsAtomicUnit=on
  ResidualCov : MATLAB Function  TreatAsAtomicUnit=on
  SOC_z : UnitDelay  InitialCondition=0.6  SampleTime=-1  HasFrameUpgradeWarning=on
  Saturation : Saturate  UpperLimit=1  LowerLimit=0
  Scope{,1..2,4..10} (10 alike) : Scope
  Scope3 : Scope  NumInputPorts=2
  "StateCorrect " : MATLAB Function  TreatAsAtomicUnit=on
  Sum : Sum  Inputs=|+-
  Sum1 : Sum  Inputs=|++
  Sum2 : Sum  Inputs=|++
  Sum3 : Sum  Inputs=|+---
  Sum4 : Sum  Inputs=|+-
  Sum5 : Sum  Inputs=|+-
  Tapped Delay : simulink/Discrete/Tapped Delay  vinit=0.0  samptime=-1  NumDelays=20  DelayOrder=Newest  includeCurrent=on
  U1_z : UnitDelay  SampleTime=-1  HasFrameUpgradeWarning=on
  U2_z : UnitDelay  SampleTime=-1  HasFrameUpgradeWarning=on
  Unit Delay : UnitDelay  InitialCondition=3.33  SampleTime=-1  HasFrameUpgradeWarning=on
  "dOCV_LUT " : Lookup_n-D  NumberOfTableDimensions=1  BreakpointsForDimension1=SOC_bp  Table=dOCV  InternalRulePriority=Speed  RndMeth=Simplest
  minus1_U1 : Constant  Value=-1
  minus1_U2 : Constant  Value=-1
  size(C_k) : Display
  size(K) : Display
  size(P_pred) : Display
  SOC_hat : Outport
  U_hat : Outport  Port=2
  residual : Outport  Port=3
  wires:
  Gain/1 -> Sum/2
  Sum/1 -> Mux/3, Display/1, SOC_z/1, Scope1/1, "dOCV_LUT "/1, 1-D Lookup Table/1  "SOC_pred"
  U1_z/1 -> Gain1/1
  Gain1/1 -> Sum1/1
  Gain2/1 -> Sum1/2
  Sum1/1 -> Sum3/3, Mux/1  "U1_pred"
  Sum2/1 -> Mux/2, Sum3/4  "U2_pred"
  Gain4/1 -> Sum2/2
  U2_z/1 -> Gain3/1
  Gain3/1 -> Sum2/1
  1-D Lookup Table/1 -> Sum3/1  "OCV_pred"
  Gain5/1 -> Sum3/2
  Sum3/1 -> Unit Delay/1  "U_hat_raw"
  Unit Delay/1 -> Scope3/1, Sum4/2  "U_hat"
  Sum4/1 -> Scope5/1, Display1/1, Tapped Delay/1, "StateCorrect "/3(res)  "residual"
  "dOCV_LUT "/1 -> Scope/1, "C_k "/1  "dOCV"
  minus1_U1/1 -> "C_k "/2
  minus1_U2/1 -> "C_k "/3
  I_k/1 -> Gain4/1, Gain2/1, Gain5/1, Gain/1
  P_z/1 -> P_predict/1(P)  "Pₖ₋₁."
  P_predict/1(Pp) -> "P_update "/1(Pp), size(P_pred)/1, R_update/3(Pp), KalmanGain/1(Pp)
  "C_k "/1 -> size(C_k)/1, "P_update "/3(C), KalmanGain/2(C), R_update/2(C)
  Constant1/1 -> A_matrix/1(a1)
  Constant2/1 -> A_matrix/2(a2)
  A_matrix/1(A) -> P_predict/2(A)
  Q_update/1(Qk) -> Scope7/1, P_predict/3(Q)
  KalmanGain/1(K) -> "StateCorrect "/2(K), "P_update "/2(K), size(K)/1  "K"
  Mux/1 -> "StateCorrect "/1(x_pred)  "x_pred"
  "StateCorrect "/1(x_hat) -> Demux/1  "x_hat   (3×1)"
  Demux/1 -> U1_z/1  "U1_hat"
  Demux/2 -> U2_z/1  "U2_hat"
  Demux/3 -> Saturation/1, Scope4/1, SOC_hat/1  "SOC_hat"
  Tapped Delay/1 -> ResidualCov/1(mu)
  ResidualCov/1(F) -> Q_update/1(F), R_update/1(F)  "F_k"
  R_update/1(Rk) -> KalmanGain/3(R), Scope6/1  "R_k"
  "P_update "/1(Pk) -> Scope2/1, P_z/1  "P_k"
  SOC_z/1 -> Scope8/1, Sum/1
  y_k/1 -> Sum5/1, Scope3/2, Sum4/1
  Sum5/1 -> Gain6/1  "residual"
  From/1 -> Scope9/1, U_hat/1, Sum5/2
  Gain6/1 -> residual/1, Scope10/1

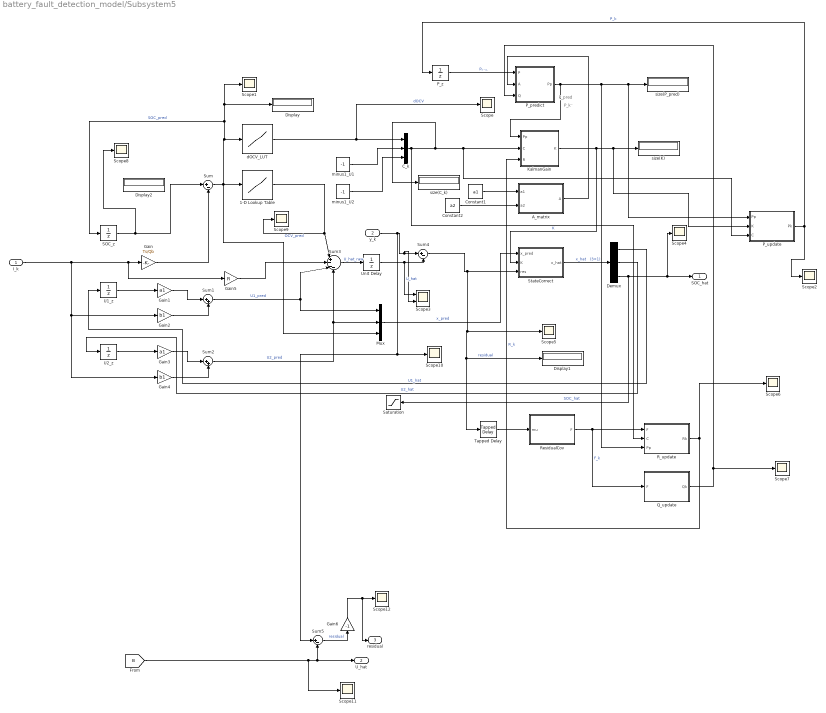
== system battery_fault_detection_model/Subsystem5 ==
  note: P_pred
  note: P_k⁻
  I_k : Inport
  y_k : Inport  Port=2
  1-D Lookup Table : Lookup_n-D  NumberOfTableDimensions=1  BreakpointsForDimension1=SOC_bp  Table=OCV  InternalRulePriority=Speed  RndMeth=Simplest
  A_matrix : MATLAB Function  TreatAsAtomicUnit=on
  "C_k " : Mux  Inputs=3
  Constant1 : Constant  Value=a1
  Constant2 : Constant  Value=a2
  Demux : Demux  Outputs=3
  Display : Display
  Display1 : Display
  Display2 : Display
  Gain : Gain  Gain=Ts/Qb
  Gain1 : Gain  Gain=a1
  Gain2 : Gain  Gain=b1
  Gain3 : Gain  Gain=a1
  Gain4 : Gain  Gain=b1
  Gain5 : Gain  Gain=R
  Gain6 : Gain  Gain=-1
  KalmanGain : MATLAB Function  TreatAsAtomicUnit=on
  Mux : Mux  Inputs=3
  P_predict : MATLAB Function  TreatAsAtomicUnit=on
  "P_update " : MATLAB Function  TreatAsAtomicUnit=on
  P_z : UnitDelay  InitialCondition=P0  SampleTime=-1  HasFrameUpgradeWarning=on
  Q_update : MATLAB Function  TreatAsAtomicUnit=on
  R_update : MATLAB Function  TreatAsAtomicUnit=on
  ResidualCov : MATLAB Function  TreatAsAtomicUnit=on
  SOC_z : UnitDelay  InitialCondition=0.6  SampleTime=-1  HasFrameUpgradeWarning=on
  Saturation : Saturate  UpperLimit=1  LowerLimit=0
  Scope{,1..2,4..12} (12 alike) : Scope
  Scope3 : Scope  NumInputPorts=2
  "StateCorrect " : MATLAB Function  TreatAsAtomicUnit=on
  Sum : Sum  Inputs=|+-
  Sum1 : Sum  Inputs=|++
  Sum2 : Sum  Inputs=|++
  Sum3 : Sum  Inputs=|+---
  Sum4 : Sum  Inputs=|+-
  Sum5 : Sum  Inputs=|+-
  Tapped Delay : simulink/Discrete/Tapped Delay  vinit=0.0  samptime=-1  NumDelays=20  DelayOrder=Newest  includeCurrent=on
  U1_z : UnitDelay  SampleTime=-1  HasFrameUpgradeWarning=on
  U2_z : UnitDelay  SampleTime=-1  HasFrameUpgradeWarning=on
  Unit Delay : UnitDelay  InitialCondition=3.32  SampleTime=-1  HasFrameUpgradeWarning=on
  "dOCV_LUT " : Lookup_n-D  NumberOfTableDimensions=1  BreakpointsForDimension1=SOC_bp  Table=dOCV  InternalRulePriority=Speed  RndMeth=Simplest
  minus1_U1 : Constant  Value=-1
  minus1_U2 : Constant  Value=-1
  size(C_k) : Display
  size(K) : Display
  size(P_pred) : Display
  SOC_hat : Outport
  U_hat : Outport  Port=2
  residual : Outport  Port=3
  wires:
  Gain/1 -> Sum/2
  Sum/1 -> Mux/3, SOC_z/1, Display/1, Scope1/1, "dOCV_LUT "/1, 1-D Lookup Table/1  "SOC_pred"
  U1_z/1 -> Gain1/1
  Gain1/1 -> Sum1/1
  Gain2/1 -> Sum1/2
  Sum1/1 -> Sum3/3, Mux/1  "U1_pred"
  Sum2/1 -> Mux/2, Sum3/4  "U2_pred"
  Gain4/1 -> Sum2/2
  U2_z/1 -> Gain3/1
  Gain3/1 -> Sum2/1
  1-D Lookup Table/1 -> Scope9/1, Sum3/1  "OCV_pred"
  Gain5/1 -> Sum3/2
  Sum3/1 -> Unit Delay/1  "U_hat_raw"
  Unit Delay/1 -> Scope3/1, Sum4/2  "U_hat"
  Sum4/1 -> Scope5/1, Display1/1, Tapped Delay/1, "StateCorrect "/3(res)  "residual"
  "dOCV_LUT "/1 -> Scope/1, "C_k "/1  "dOCV"
  minus1_U1/1 -> "C_k "/2
  minus1_U2/1 -> "C_k "/3
  I_k/1 -> Gain4/1, Gain2/1, Gain5/1, Gain/1
  P_z/1 -> P_predict/1(P)  "Pₖ₋₁."
  P_predict/1(Pp) -> "P_update "/1(Pp), size(P_pred)/1, R_update/3(Pp), KalmanGain/1(Pp)
  "C_k "/1 -> size(C_k)/1, "P_update "/3(C), KalmanGain/2(C), R_update/2(C)
  Constant1/1 -> A_matrix/1(a1)
  Constant2/1 -> A_matrix/2(a2)
  A_matrix/1(A) -> P_predict/2(A)
  Q_update/1(Qk) -> Scope7/1, P_predict/3(Q)
  KalmanGain/1(K) -> "StateCorrect "/2(K), "P_update "/2(K), size(K)/1  "K"
  Mux/1 -> "StateCorrect "/1(x_pred)  "x_pred"
  "StateCorrect "/1(x_hat) -> Demux/1  "x_hat   (3×1)"
  Demux/1 -> U1_z/1  "U1_hat"
  Demux/2 -> U2_z/1  "U2_hat"
  Demux/3 -> Saturation/1, Scope4/1, SOC_hat/1  "SOC_hat"
  Tapped Delay/1 -> ResidualCov/1(mu)
  ResidualCov/1(F) -> Q_update/1(F), R_update/1(F)  "F_k"
  R_update/1(Rk) -> KalmanGain/3(R), Scope6/1  "R_k"
  "P_update "/1(Pk) -> P_z/1, Scope2/1  "P_k"
  SOC_z/1 -> Scope8/1, Sum/1
  Sum5/1 -> Gain6/1  "residual"
  y_k/1 -> Scope10/1, Sum5/1, Scope3/2, Sum4/1
  [B] -> Scope11/1, U_hat/1, Sum5/2
  Gain6/1 -> residual/1, Scope12/1

== matlab function battery_fault_detection_model/Subsystem1/P_update  ==
  data: Pp input; Pk output; K input; C input
function Pk = P_update(Pp, K, C)
% Updated covariance: Pk = (I - K*C) * Pp
C = reshape(C,1,3);
I = eye(3);
Pk = (I - K*C) * Pp;
end

== matlab function battery_fault_detection_model/Subsystem1/Q_update ==
  data: F input; Qk output
function Qk = Q_update(F)
Qk = diag([0, 0, F]);   % 3×3 matrix
end

== matlab function battery_fault_detection_model/Subsystem5/P_predict ==
  data: P input; Pp output; A input; Q input
function Pp = P_predict(P, A, Q)
Pp = A*P*A' + Q;
end

== matlab function battery_fault_detection_model/Subsystem1/R_update ==
  data: F input; Rk output; C input; Pp input
function Rk = R_update(F, C, Pp)
C = reshape(C,1,3);
Rk = F + C*Pp*C';
end

== matlab function battery_fault_detection_model/Subsystem1/ResidualCov ==
  data: mu input; F output
function F = ResidualCov(mu)
mu = mu(:);              % force column vector
N  = length(mu);
F  = sum(mu.^2)/(N-1);   % scalar variance
end

== matlab function battery_fault_detection_model/Subsystem1/StateCorrect  ==
  data: x_pred input; x_hat output; K input; res input
function x_hat = StateCorrect(x_pred, K, res)
x_hat = x_pred + K * res;
end

== matlab function battery_fault_detection_model/Subsystem2/A_matrix ==
  data: a1 input; A output; a2 input
function A = A_matrix(a1, a2)
A = [a1 0  0;
     0  a2 0;
     0  0  1];
end

== matlab function battery_fault_detection_model/Subsystem2/KalmanGain ==
  data: Pp input; K output; C input; R input
function K = KalmanGain(Pp, C, R)
% Force dimensions explicitly
C = reshape(C, 1, 3);   % 1×3 row vector

S = C*Pp*C' + R;        % scalar
K = (Pp*C') / S;        % 3×1
end

== matlab function battery_fault_detection_model/Subsystem2/P_predict ==
  data: P input; Pp output; A input; Q input
function Pp = P_predict(P, A, Q)
Pp = A*P*A' + Q;
end

== matlab function battery_fault_detection_model/Subsystem2/P_update  ==
  data: Pp input; Pk output; K input; C input
function Pk = P_update(Pp, K, C)
% Updated covariance: Pk = (I - K*C) * Pp
C = reshape(C,1,3);
I = eye(3);
Pk = (I - K*C) * Pp;
end

== matlab function battery_fault_detection_model/Subsystem2/Q_update ==
  data: F input; Qk output
function Qk = Q_update(F)
Qk = diag([0, 0, F]);   % 3×3 matrix
end

== matlab function battery_fault_detection_model/Subsystem2/R_update ==
  data: F input; Rk output; C input; Pp input
function Rk = R_update(F, C, Pp)
C = reshape(C,1,3);
Rk = F + C*Pp*C';
end

== matlab function battery_fault_detection_model/Subsystem2/ResidualCov ==
  data: mu input; F output
function F = ResidualCov(mu)
mu = mu(:);              % force column vector
N  = length(mu);
F  = sum(mu.^2)/(N-1);   % scalar variance
end

== matlab function battery_fault_detection_model/Subsystem2/StateCorrect  ==
  data: x_pred input; x_hat output; K input; res input
function x_hat = StateCorrect(x_pred, K, res)
x_hat = x_pred + K * res;
end

== matlab function battery_fault_detection_model/Subsystem5/A_matrix ==
  data: a1 input; A output; a2 input
function A = A_matrix(a1, a2)
A = [a1 0  0;
     0  a2 0;
     0  0  1];
end

== matlab function battery_fault_detection_model/Subsystem3/A_matrix ==
  data: a1 input; A output; a2 input
function A = A_matrix(a1, a2)
A = [a1 0  0;
     0  a2 0;
     0  0  1];
end

== matlab function battery_fault_detection_model/Subsystem3/KalmanGain ==
  data: Pp input; K output; C input; R input
function K = KalmanGain(Pp, C, R)
% Force dimensions explicitly
C = reshape(C, 1, 3);   % 1×3 row vector

S = C*Pp*C' + R;        % scalar
K = (Pp*C') / S;        % 3×1
end

== matlab function battery_fault_detection_model/Subsystem3/P_predict ==
  data: P input; Pp output; A input; Q input
function Pp = P_predict(P, A, Q)
Pp = A*P*A' + Q;
end

== matlab function battery_fault_detection_model/Subsystem3/P_update  ==
  data: Pp input; Pk output; K input; C input
function Pk = P_update(Pp, K, C)
% Updated covariance: Pk = (I - K*C) * Pp
C = reshape(C,1,3);
I = eye(3);
Pk = (I - K*C) * Pp;
end

== matlab function battery_fault_detection_model/Subsystem3/Q_update ==
  data: F input; Qk output
function Qk = Q_update(F)
Qk = diag([0, 0, F]);   % 3×3 matrix
end

== matlab function battery_fault_detection_model/Subsystem3/R_update ==
  data: F input; Rk output; C input; Pp input
function Rk = R_update(F, C, Pp)
C = reshape(C,1,3);
Rk = F + C*Pp*C';
end

== matlab function battery_fault_detection_model/Subsystem3/ResidualCov ==
  data: mu input; F output
function F = ResidualCov(mu)
mu = mu(:);              % force column vector
N  = length(mu);
F  = sum(mu.^2)/(N-1);   % scalar variance
end

== matlab function battery_fault_detection_model/Subsystem3/StateCorrect  ==
  data: x_pred input; x_hat output; K input; res input
function x_hat = StateCorrect(x_pred, K, res)
x_hat = x_pred + K * res;
end

== matlab function battery_fault_detection_model/Subsystem4/A_matrix ==
  data: a1 input; A output; a2 input
function A = A_matrix(a1, a2)
A = [a1 0  0;
     0  a2 0;
     0  0  1];
end

== matlab function battery_fault_detection_model/Subsystem4/KalmanGain ==
  data: Pp input; K output; C input; R input
function K = KalmanGain(Pp, C, R)
% Force dimensions explicitly
C = reshape(C, 1, 3);   % 1×3 row vector

S = C*Pp*C' + R;        % scalar
K = (Pp*C') / S;        % 3×1
end

== matlab function battery_fault_detection_model/Subsystem5/KalmanGain ==
  data: Pp input; K output; C input; R input
function K = KalmanGain(Pp, C, R)
% Force dimensions explicitly
C = reshape(C, 1, 3);   % 1×3 row vector

S = C*Pp*C' + R;        % scalar
K = (Pp*C') / S;        % 3×1
end

== matlab function battery_fault_detection_model/Subsystem4/P_predict ==
  data: P input; Pp output; A input; Q input
function Pp = P_predict(P, A, Q)
Pp = A*P*A' + Q;
end

== matlab function battery_fault_detection_model/Subsystem4/P_update  ==
  data: Pp input; Pk output; K input; C input
function Pk = P_update(Pp, K, C)
% Updated covariance: Pk = (I - K*C) * Pp
C = reshape(C,1,3);
I = eye(3);
Pk = (I - K*C) * Pp;
end

== matlab function battery_fault_detection_model/Subsystem4/Q_update ==
  data: F input; Qk output
function Qk = Q_update(F)
Qk = diag([0, 0, F]);   % 3×3 matrix
end

== matlab function battery_fault_detection_model/Subsystem4/R_update ==
  data: F input; Rk output; C input; Pp input
function Rk = R_update(F, C, Pp)
C = reshape(C,1,3);
Rk = F + C*Pp*C';
end

== matlab function battery_fault_detection_model/Subsystem4/ResidualCov ==
  data: mu input; F output
function F = ResidualCov(mu)
mu = mu(:);              % force column vector
N  = length(mu);
F  = sum(mu.^2)/(N-1);   % scalar variance
end

== matlab function battery_fault_detection_model/Subsystem4/StateCorrect  ==
  data: x_pred input; x_hat output; K input; res input
function x_hat = StateCorrect(x_pred, K, res)
x_hat = x_pred + K * res;
end

== matlab function battery_fault_detection_model/MATLAB Function1 ==
  data: r input; s output
function s = loglikelihood_step(r)
sigma = 0.002;   % start here
s = (r.^2) / (2*sigma^2);
end

== matlab function battery_fault_detection_model/cusum_update  ==
  data: r input; S output
function S = cusum_step(r)

% r = residual (already filtered if you want)

persistent Sk
if isempty(Sk)
    Sk = 0;
end

% === TUNED PARAMETERS (WORKING RANGE) ===
h = 0.02;     % drift (must be SMALLER than fault bias)
Smax = 1e6;   % prevent overflow (safety)

% === ONE-SIDED CUSUM ===
Sk = max(0, Sk + r - h);

% Saturation (numerical safety)
Sk = min(Sk, Smax);

S = Sk;
end

== matlab function battery_fault_detection_model/fault_flag ==
  data: d_umax input; fault output; d_umin input; d_ui input
function fault = fault_isolation(d_umax, d_umin, d_ui)
if d_umax && d_umin
    fault = 2;   % current sensor fault
elseif d_umax
    fault = 3;   % voltage sensor fault (max cell)
elseif d_umin
    fault = 4;   % voltage sensor fault (min cell)
else
    fault = 0;   % healthy
end
end

== matlab function battery_fault_detection_model/Subsystem5/StateCorrect  ==
  data: x_pred input; x_hat output; K input; res input
function x_hat = StateCorrect(x_pred, K, res)
x_hat = x_pred + K * res;
end

== matlab function battery_fault_detection_model/Subsystem5/ResidualCov ==
  data: mu input; F output
function F = ResidualCov(mu)
mu = mu(:);              % force column vector
N  = length(mu);
F  = sum(mu.^2)/(N-1);   % scalar variance
end

== matlab function battery_fault_detection_model/Subsystem5/R_update ==
  data: F input; Rk output; C input; Pp input
function Rk = R_update(F, C, Pp)
C = reshape(C,1,3);
Rk = F + C*Pp*C';
end

== matlab function battery_fault_detection_model/Subsystem5/Q_update ==
  data: F input; Qk output
function Qk = Q_update(F)
Qk = diag([0, 0, F]);   % 3×3 matrix
end

== matlab function battery_fault_detection_model/Subsystem5/P_update  ==
  data: Pp input; Pk output; K input; C input
function Pk = P_update(Pp, K, C)
% Updated covariance: Pk = (I - K*C) * Pp
C = reshape(C,1,3);
I = eye(3);
Pk = (I - K*C) * Pp;
end

== matlab function battery_fault_detection_model/Subsystem1/A_matrix ==
  data: a1 input; A output; a2 input
function A = A_matrix(a1, a2)
A = [a1 0  0;
     0  a2 0;
     0  0  1];
end

== matlab function battery_fault_detection_model/Subsystem1/KalmanGain ==
  data: Pp input; K output; C input; R input
function K = KalmanGain(Pp, C, R)
% Force dimensions explicitly
C = reshape(C, 1, 3);   % 1×3 row vector

S = C*Pp*C' + R;        % scalar
K = (Pp*C') / S;        % 3×1
end

== matlab function battery_fault_detection_model/Subsystem1/P_predict ==
  data: P input; Pp output; A input; Q input
function Pp = P_predict(P, A, Q)
Pp = A*P*A' + Q;
end
